simulink model "marsrover_visualisation"  (R2015b)
settings: Solver=VariableStepAuto  StartTime=0.0  StopTime=10.0  RelTol=1e-3
settings Model: Creator=akash  LastModifiedBy=akash

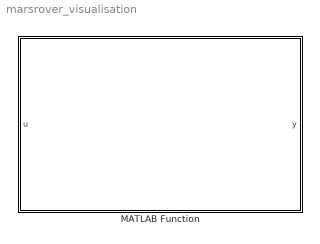
== system marsrover_visualisation ==
  MATLAB Function : MATLAB Function  TreatAsAtomicUnit=on

== matlab function marsrover_visualisation/MATLAB Function ==
  data: u input; y output
function y = fcn(u)
%#codegen

y = u;
